simulink model "RNN_Activation"  (R2020b)
settings: Solver=VariableStepAuto  StartTime=0.0  StopTime=10.0  RelTol=1e-3
settings Model: Creator=chank  LastModifiedBy=chank

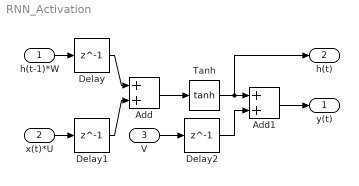
== system RNN_Activation ==
  h(t-1)*W : Inport  OutDataTypeStr=single
  x(t)*U : Inport  Port=2  OutDataTypeStr=single
  V : Inport  Port=3  OutDataTypeStr=single
  Add : Sum
  Add1 : Sum
  Delay : Delay  DelayLength=1
  Delay1 : Delay  DelayLength=1
  Delay2 : Delay  DelayLength=1
  Tanh : Trigonometry  Operator=tanh
  y(t) : Outport
  h(t) : Outport  Port=2
  wires:
  Add/1 -> Tanh/1
  Tanh/1 -> h(t)/1, Add1/1
  Add1/1 -> y(t)/1
  h(t-1)*W/1 -> Delay/1
  Delay/1 -> Add/1
  x(t)*U/1 -> Delay1/1
  Delay1/1 -> Add/2
  V/1 -> Delay2/1
  Delay2/1 -> Add1/2
